simulink model "sim2"  (R2020b)
settings: Solver=VariableStepAuto  StartTime=0.0  StopTime=300  RelTol=1e-3
undefined symbols (not defined in the file): h, SP, T, tau
settings Model: Creator=48576  LastModifiedBy=48576

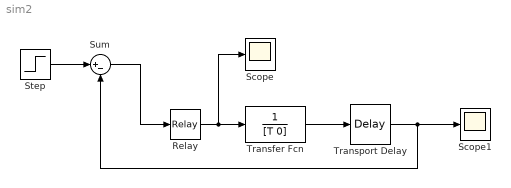
== system sim2 ==
  Relay : Relay  OnSwitchValue=h  OffSwitchValue=-h  OffOutputValue=-1
  Scope : Scope
  Scope1 : Scope
  Step : Step  After=SP  SampleTime=0
  Sum : Sum  Inputs=|+-
  Transfer Fcn : TransferFcn  Denominator=[T 0]
  Transport Delay : TransportDelay  DelayTime=tau  PadeOrder=10
  wires:
  Transport Delay/1 -> Sum/2, Scope1/1
  Relay/1 -> Scope/1, Transfer Fcn/1
  Sum/1 -> Relay/1
  Step/1 -> Sum/1
  Transfer Fcn/1 -> Transport Delay/1
